simulink model "vizTest"  (R2012b)
settings: Solver=FixedStepDiscrete  StartTime=0.0  StopTime=10.0  FixedStep=0.001  RelTol=1e-3
undefined symbols (not defined in the file): clickHoldTime, clickPercentage, clickSource, cursorConstants, cursorDiameter, expRandBinSize, expRandMax, expRandMin, expRandMu, failurePenalty, gain, gloveBias, gloveIndices, gloveThreshold, hmmClickLikelihoodThreshold, holdTime, initialInput, inputType, mouseOffset, numTargets, numTrials, pbData, randomSeed, recenterDelay, recenterOnFail, recenterOnSuccess, showNeuralCursor, showScores, stopOnClick, targetDiameter, targetInds, taskType, trialsPerScore, trialTimeout, useRandomDelay, workspaceX, workspaceY
libraries: simulink x1, xpclib x1
settings Model: BufferReuse=off  Creator=gilja  LastModifiedBy=nptl
settings SolverCC: EnableConcurrentExecution=on  ConcurrentTasks=on
settings DataIOCC: SaveOutput=off  SignalLogging=off  SaveTime=off
settings OptimizationCC: InlineParams=on  InlineInvariantSignals=on  OptimizeBlockIOStorage=off  BufferReuse=off  ExpressionFolding=off  LocalBlockOutputs=off  SimCompilerOptimization=On
settings DebuggingCC: UnderspecifiedInitializationDetection=Simplified
settings HardwareCC: ProdIntDivRoundTo=Zero  ProdEndianess=LittleEndian  ProdHWDeviceType=Generic->32-bit x86 compatible
settings ModelReferenceCC: ModelReferenceNumInstancesAllowed=Single  ModelReferenceMinAlgLoopOccurrences=on
settings RTWCC: SystemTargetFile=xpctarget.tlc  TemplateMakefile=xpc_default_tmf  Description=xPC Target  ProcessScript=xpctarget_make_rtw_hook  RTWCompilerOptimization=On
settings CodeAppCC: MaxIdLength=62
settings xpcTargetCC: TargetFcnLib=ansi_tfl_table_tmw.mat  CodeReplacementLibrary=XPC_BLAS  ParMdlRefBuildCompliant=on  ConcurrentExecutionCompliant=on  CombineSignalStateStructs=off  GRTInterface=on  xPCTaskExecutionProfile=on  xPCRL32EventNumber=5000  xPCisDownloadable=off  xPCLoadParamSetFile=off  xPCConcurrentTasks=off  xPCEnableSFAnimation=off

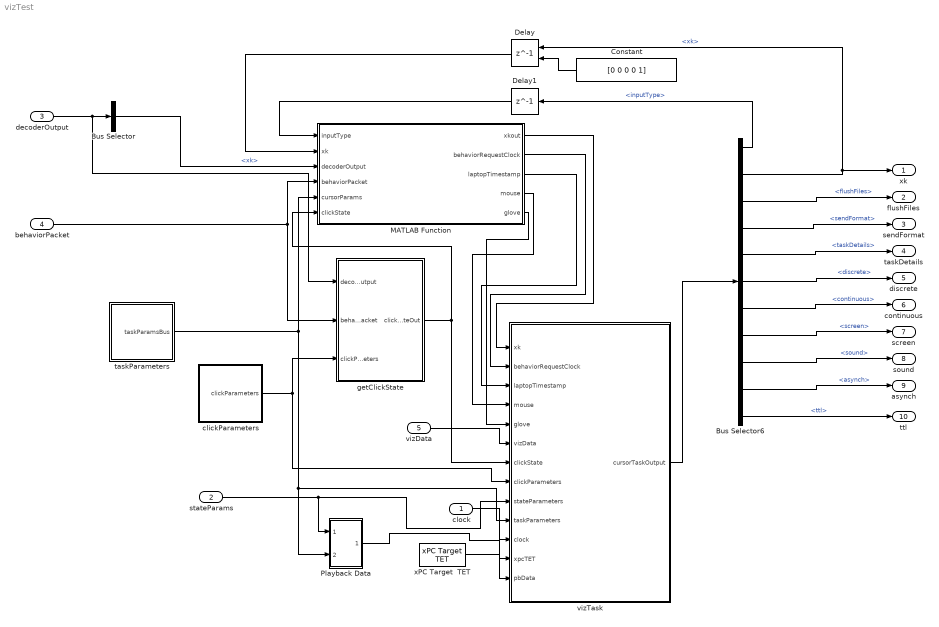
== system vizTest ==
  clock : Inport  OutDataTypeStr=uint32
  stateParams : Inport  Port=2  OutDataTypeStr=Bus: stateParams
  decoderOutput : Inport  Port=3  OutDataTypeStr=Bus: decoderOutput
  behaviorPacket : Inport  Port=4  OutDataTypeStr=Bus: behaviorPacketBus
  vizData : Inport  Port=5  OutDataTypeStr=Bus: peripheralData
  Bus Selector : BusSelector  OutputSignals=xk
  Bus Selector6 : BusSelector  OutputSignals=inputType,xk,flushFiles,sendFormat,taskDetails,discrete,continuous,screen,sound,asynch,ttl
  Constant : Constant  Value=[0 0 0 0 1]
  Delay : Delay  DelayLength=1  InitialConditionSource=Input port  InitialCondition=0
      settings: InputPortMap=u0,p4
  Delay1 : Delay  DelayLength=1  InitialCondition=0
  MATLAB Function : MATLAB Function  TreatAsAtomicUnit=on
  Playback Data : Subsystem
  clickParameters : Subsystem
  getClickState : MATLAB Function  TreatAsAtomicUnit=on
  taskParameters : Subsystem
  vizTask : MATLAB Function  TreatAsAtomicUnit=on
  "xPC Target  TET " : xpclib/Misc./xPC Target  TET   ts=0.001
  xk : Outport
  flushFiles : Outport  Port=2
  sendFormat : Outport  Port=3
  taskDetails : Outport  Port=4  OutDataTypeStr=Bus: fileLoggerFormat  BusOutputAsStruct=on
  discrete : Outport  Port=5  OutDataTypeStr=Bus: fileLoggerFormatAndData  BusOutputAsStruct=on
  continuous : Outport  Port=6  OutDataTypeStr=Bus: fileLoggerFormatAndData  BusOutputAsStruct=on
  screen : Outport  Port=7  OutDataTypeStr=Bus: fileLoggerFormatAndData  BusOutputAsStruct=on
  sound : Outport  Port=8  OutDataTypeStr=Bus: fileLoggerFormatAndData  BusOutputAsStruct=on
  asynch : Outport  Port=9  OutDataTypeStr=Bus: fileLoggerFormatAndData  BusOutputAsStruct=on
  ttl : Outport  Port=10  OutDataTypeStr=double  BusOutputAsStruct=on
  wires:
  clock/1 -> vizTask/11(clock)
  taskParameters/1(taskParamsBus) -> MATLAB Function/5(cursorParams), vizTask/10(taskParameters), Playback Data/2(cursorParams)
  "xPC Target  TET "/1 -> vizTask/12(xpcTET)
  stateParams/1 -> vizTask/9(stateParameters), Playback Data/1(stateParams)
  vizTask/1(cursorTaskOutput) -> Bus Selector6/1
  Bus Selector6/2 -> Delay/1, xk/1  "<xk>"
  Bus Selector6/3 -> flushFiles/1  "<flushFiles>"
  Bus Selector6/4 -> sendFormat/1  "<sendFormat>"
  Bus Selector6/6 -> discrete/1  "<discrete>"
  Bus Selector6/7 -> continuous/1  "<continuous>"
  Bus Selector6/5 -> taskDetails/1  "<taskDetails>"
  vizData/1 -> vizTask/6(vizData)
  MATLAB Function/1(xkout) -> vizTask/1(xk)
  Bus Selector6/8 -> screen/1  "<screen>"
  Delay/1 -> MATLAB Function/2(xk)
  MATLAB Function/2(behaviorRequestClock) -> vizTask/2(behaviorRequestClock)
  MATLAB Function/3(laptopTimestamp) -> vizTask/3(laptopTimestamp)
  MATLAB Function/4(mouse) -> vizTask/4(mouse)
  Bus Selector6/1 -> Delay1/1  "<inputType>"
  Delay1/1 -> MATLAB Function/1(inputType)
  Constant/1 -> Delay/2
  Playback Data/1(pbData) -> vizTask/13(pbData)
  behaviorPacket/1 -> MATLAB Function/4(behaviorPacket), getClickState/2(behaviorPacket)
  clickParameters/1(clickParameters) -> getClickState/3(clickParameters), vizTask/8(clickParameters)
  getClickState/1(clickStateOut) -> vizTask/7(clickState), MATLAB Function/6(clickState)
  MATLAB Function/5(glove) -> vizTask/5(glove)
  decoderOutput/1 -> getClickState/1(decoderOutput), Bus Selector/1
  Bus Selector/1 -> MATLAB Function/3(decoderOutput)  "<xk>"
  Bus Selector6/11 -> ttl/1  "<ttl>"
  Bus Selector6/9 -> sound/1  "<sound>"
  Bus Selector6/10 -> asynch/1  "<asynch>"

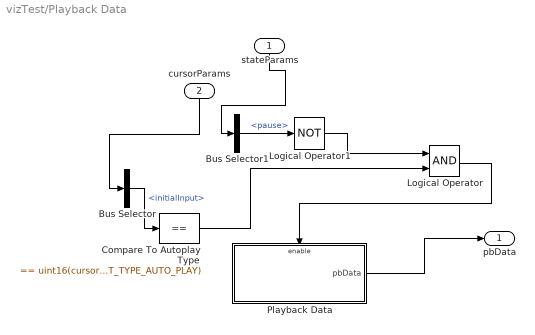
== system vizTest/Playback Data ==
  stateParams : Inport
  cursorParams : Inport  Port=2
  Bus Selector : BusSelector  OutputSignals=initialInput
  Bus Selector1 : BusSelector  OutputSignals=pause
  Compare To Autoplay Type : simulink/Logic and Bit Operations/Compare To Constant  relop===  const=uint16(cursorConstants.INPUT_TYPE_AUTO_PLAY)  OutDataTypeStr=boolean
  Logical Operator : Logic  AllPortsSameDT=off  OutDataTypeStr=boolean
  Logical Operator1 : Logic  Operator=NOT  AllPortsSameDT=off  OutDataTypeStr=boolean
  Playback Data : Subsystem
  pbData : Outport
  wires:
  Logical Operator/1 -> Playback Data/Enable
  Playback Data/1(pbData) -> pbData/1
  stateParams/1 -> Bus Selector1/1
  cursorParams/1 -> Bus Selector/1
  Bus Selector1/1 -> Logical Operator1/1  "<pause>"
  Bus Selector/1 -> Compare To Autoplay Type/1  "<initialInput>"
  Compare To Autoplay Type/1 -> Logical Operator/2
  Logical Operator1/1 -> Logical Operator/1

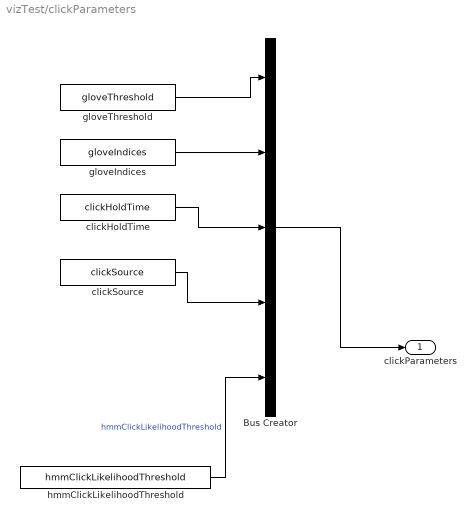
== system vizTest/clickParameters ==
  Bus Creator : BusCreator  Inputs=5  OutDataTypeStr=Bus: clickParametersBus  NonVirtualBus=on
  clickHoldTime : Constant  Value=clickHoldTime
  clickSource : Constant  Value=clickSource
  gloveIndices : Constant  Value=gloveIndices
  gloveThreshold : Constant  Value=gloveThreshold
  hmmClickLikelihoodThreshold : Constant  Value=hmmClickLikelihoodThreshold  VectorParams1D=off
  clickParameters : Outport
  wires:
  Bus Creator/1 -> clickParameters/1
  gloveThreshold/1 -> Bus Creator/1
  gloveIndices/1 -> Bus Creator/2
  clickHoldTime/1 -> Bus Creator/3
  clickSource/1 -> Bus Creator/4
  hmmClickLikelihoodThreshold/1 -> Bus Creator/5  "hmmClickLikelihoodThreshold"

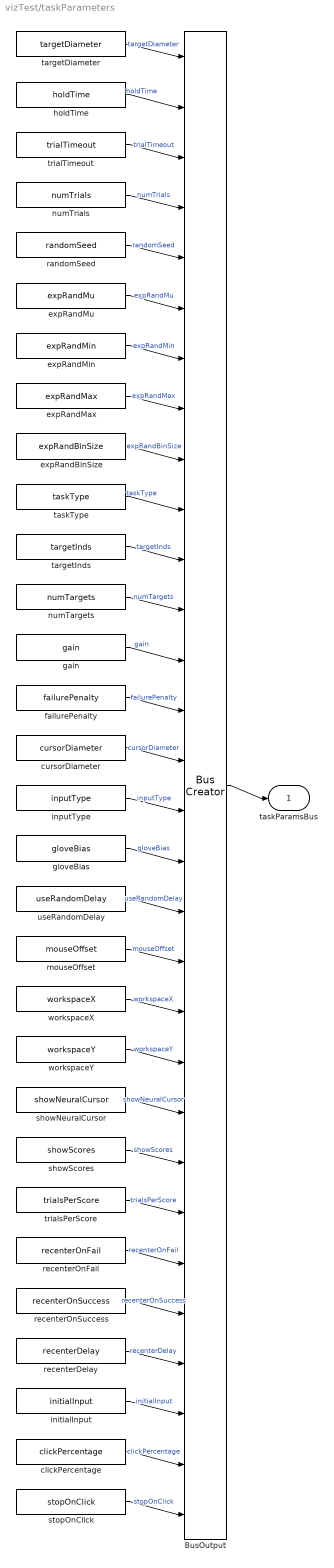
== system vizTest/taskParameters ==
  BusOutput : BusCreator  Inputs=targetDiameter,holdTime,trialTimeout,numTrials,randomSeed,expRandMu,expRandMin,expRandMax,expRandBinSize,taskType,targetInds,numTargets,gain,failurePenalty,cursorDiameter,inputType,gloveBias,useRandomDelay,mouseOffset,workspaceX,workspaceY,showNeuralCursor,showScores,trialsPerScore,recenterOnFail,recenterOnSuccess,recenterDelay,initialInput,clickPercentage,stopOnClick  OutDataTypeStr=Bus: taskParamsBus
  clickPercentage : Constant  Value=clickPercentage
  cursorDiameter : Constant  Value=cursorDiameter
  expRandBinSize : Constant  Value=expRandBinSize
  expRandMax : Constant  Value=expRandMax
  expRandMin : Constant  Value=expRandMin
  expRandMu : Constant  Value=expRandMu
  failurePenalty : Constant  Value=failurePenalty
  gain : Constant  Value=gain
  gloveBias : Constant  Value=gloveBias
  holdTime : Constant  Value=holdTime
  initialInput : Constant  Value=initialInput
  inputType : Constant  Value=inputType
  mouseOffset : Constant  Value=mouseOffset
  numTargets : Constant  Value=numTargets
  numTrials : Constant  Value=numTrials
  randomSeed : Constant  Value=randomSeed
  recenterDelay : Constant  Value=recenterDelay
  recenterOnFail : Constant  Value=recenterOnFail
  recenterOnSuccess : Constant  Value=recenterOnSuccess
  showNeuralCursor : Constant  Value=showNeuralCursor
  showScores : Constant  Value=showScores
  stopOnClick : Constant  Value=stopOnClick
  targetDiameter : Constant  Value=targetDiameter
  targetInds : Constant  Value=targetInds
  taskType : Constant  Value=taskType
  trialTimeout : Constant  Value=trialTimeout
  trialsPerScore : Constant  Value=trialsPerScore
  useRandomDelay : Constant  Value=useRandomDelay
  workspaceX : Constant  Value=workspaceX
  workspaceY : Constant  Value=workspaceY
  taskParamsBus : Outport
  wires:
  targetDiameter/1 -> BusOutput/1  "targetDiameter"
  holdTime/1 -> BusOutput/2  "holdTime"
  trialTimeout/1 -> BusOutput/3  "trialTimeout"
  numTrials/1 -> BusOutput/4  "numTrials"
  randomSeed/1 -> BusOutput/5  "randomSeed"
  expRandMu/1 -> BusOutput/6  "expRandMu"
  expRandMin/1 -> BusOutput/7  "expRandMin"
  expRandMax/1 -> BusOutput/8  "expRandMax"
  expRandBinSize/1 -> BusOutput/9  "expRandBinSize"
  taskType/1 -> BusOutput/10  "taskType"
  targetInds/1 -> BusOutput/11  "targetInds"
  numTargets/1 -> BusOutput/12  "numTargets"
  gain/1 -> BusOutput/13  "gain"
  failurePenalty/1 -> BusOutput/14  "failurePenalty"
  cursorDiameter/1 -> BusOutput/15  "cursorDiameter"
  inputType/1 -> BusOutput/16  "inputType"
  gloveBias/1 -> BusOutput/17  "gloveBias"
  useRandomDelay/1 -> BusOutput/18  "useRandomDelay"
  mouseOffset/1 -> BusOutput/19  "mouseOffset"
  workspaceX/1 -> BusOutput/20  "workspaceX"
  workspaceY/1 -> BusOutput/21  "workspaceY"
  showNeuralCursor/1 -> BusOutput/22  "showNeuralCursor"
  showScores/1 -> BusOutput/23  "showScores"
  trialsPerScore/1 -> BusOutput/24  "trialsPerScore"
  recenterOnFail/1 -> BusOutput/25  "recenterOnFail"
  recenterOnSuccess/1 -> BusOutput/26  "recenterOnSuccess"
  recenterDelay/1 -> BusOutput/27  "recenterDelay"
  initialInput/1 -> BusOutput/28  "initialInput"
  clickPercentage/1 -> BusOutput/29  "clickPercentage"
  stopOnClick/1 -> BusOutput/30  "stopOnClick"
  BusOutput/1 -> taskParamsBus/1

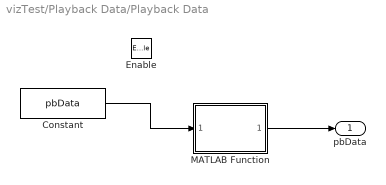
== system vizTest/Playback Data/Playback Data ==
  Enable : EnablePort
  Constant : Constant  Value=pbData
  MATLAB Function : MATLAB Function  TreatAsAtomicUnit=on
  pbData : Outport  InitialOutput=[0]
  wires:
  Constant/1 -> MATLAB Function/1(pbData)
  MATLAB Function/1(pbDataSelect) -> pbData/1

== matlab function vizTest/Playback Data/Playback Data/MATLAB Function ==
  data: pbData input single; pbDataSelect output single
function pbDataSelect = fcn(pbData)
%#codegen
persistent idx;

MAX_PLAYBACK_LENGTH = 300*1000;

if(isempty(idx))
    idx = 1;
end

pbDataSelect = pbData(idx, :);

if((idx < size(pbData,1)) && (idx < MAX_PLAYBACK_LENGTH))
    idx = idx + 1;
else
    pbDataSelect = single([0 -10000 -10000 -10000 -10000]);
end

== matlab function vizTest/MATLAB Function ==
  data: inputType input uint16 size=1; xk input size=[5 1]; decoderOutput input size=[5 1]; xkout output size=[5 1]; behaviorPacket input; cursorParams input; behaviorRequestClock output uint32 size=1; laptopTimestamp output uint8 size=16; mouse output int32 size=6; clickState input; glove output
function [xkout,behaviorRequestClock, laptopTimestamp, mouse, glove] = updateXk(inputType, xk, decoderOutput, behaviorPacket, cursorParams, clickState)


xkout = xk;

if ~cursorParams.stopOnClick || clickState == uint16(DiscreteStates.CLICK_IDLE) 
    switch inputType
        case cursorConstants.INPUT_TYPE_MOUSE_RELATIVE
            xkout(3) = cursorParams.gain(1).*double(behaviorPacket.mouse(1));
            xkout(4) = cursorParams.gain(2).*double(behaviorPacket.mouse(2));
        case cursorConstants.INPUT_TYPE_MOUSE_ABSOLUTE
            xkout(3) = cursorParams.gain(1).*(double(behaviorPacket.mouse(1))-double(cursorParams.mouseOffset(1))) - xk(1);
            xkout(4) = cursorParams.gain(2).*(double(behaviorPacket.mouse(2))-double(cursorParams.mouseOffset(2))) - xk(2);
        case cursorConstants.INPUT_TYPE_DECODE_V
            xkout(3) = decoderOutput(3);
            xkout(4) = decoderOutput(4);
    end
    xkout(1:2) = xkout(1:2)+xkout(3:4);
    if xkout(1) > cursorParams.workspaceX(2)
        xkout(1) = cursorParams.workspaceX(2);
        xkout(3) = 0;
    elseif xkout(1) < cursorParams.workspaceX(1)
        xkout(1) = cursorParams.workspaceX(1);
        xkout(3) = 0;
    end
    if xkout(2) > cursorParams.workspaceY(2)
        xkout(2) = cursorParams.workspaceY(2);
        xkout(4) = 0;
    elseif xkout(2) < cursorParams.workspaceY(1)
        xkout(2) = cursorParams.workspaceY(1);
        xkout(4) = 0;
    end
end
mouse = behaviorPacket.mouse(1:6);
glove = behaviorPacket.glove(1:5);
behaviorRequestClock = behaviorPacket.xpcRequestClock;
laptopTimestamp = behaviorPacket.laptopTimestamp(1:16);

end

== matlab function vizTest/vizTask ==
  data: xk input double size=[5 1]; behaviorRequestClock input uint32 size=1; laptopTimestamp input uint8 size=16; mouse input int32 size=6; glove input; vizData input Bus: peripheralData; clickState input; clickParameters input Bus: clickParametersBus; cursorTaskOutput output Bus: cursorTaskOutput; stateParameters input Bus: stateParams size=1; taskParameters input Bus: taskParamsBus; clock input; xpcTET input; pbData input single
function cursorTaskOutput  = vizTest(xk, behaviorRequestClock, laptopTimestamp, mouse, glove, vizData, clickState, clickParameters, stateParameters, taskParameters, clock, xpcTET, pbData)
%#codegen

%% CONSTANTS
TASK_NAME = 'viztest';
VERSION_ID = single(2.010);
NUM_DIMS = double(cursorConstants.NUM_DIMENSIONS);
STATEVEC_SIZE = 2*NUM_DIMS+1;
INIT_LENGTH = uint16(100); %ms
PRE_TRIAL_LENGTH = uint16(20); %ms
SCORE_LENGTH = uint16(4000); %ms
INIT_TIME = uint32(100);
CUE_LENGTH = taskParameters.holdTime;%uint16(200);
BLANK_LENGTH = uint16(800);


%% INITIALIZE CURSOR TASK OUTPUT
fileLoggerData.data = uint8(zeros(1,1400));
fileLoggerData.dataLen = uint16(0);
fileLoggerData.fileName = uint8(zeros(1,20));
fileLoggerData.send = false;

fileLoggerFormat.format = uint8(zeros(1,1400));
fileLoggerFormat.formatLen = uint16(0);
fileLoggerFormat.fileName = uint8(zeros(1,20));

fileLoggerFormatAndData.format = fileLoggerFormat;
fileLoggerFormatAndData.data = fileLoggerData;

cursorTaskOutput.flushFiles = false;
cursorTaskOutput.sendFormat = false;
cursorTaskOutput.taskDetails = fileLoggerFormat;
cursorTaskOutput.discrete = fileLoggerFormatAndData;
cursorTaskOutput.continuous = fileLoggerFormatAndData;
cursorTaskOutput.screen = fileLoggerFormatAndData;
cursorTaskOutput.sound = fileLoggerFormatAndData;
cursorTaskOutput.asynch = fileLoggerFormatAndData;
cursorTaskOutput.ttl = double(0);
cursorTaskOutput.xk = xk;
cursorTaskOutput.inputType = taskParameters.initialInput;

%% TASK DETAILS PACKET
cursorTaskOutput.taskDetails = packFileLoggerTaskDetails(TASK_NAME, VERSION_ID, ...
    'STATE_INIT', uint8(CursorStates.STATE_INIT), ...
    'STATE_PRE_TRIAL', uint8(CursorStates.STATE_PRE_TRIAL),...
    'STATE_NEW_TARGET', uint8(CursorStates.STATE_NEW_TARGET),...
    'STATE_MOVE', uint8(CursorStates.STATE_MOVE),...
    'STATE_ACQUIRE', uint8(CursorStates.STATE_ACQUIRE),...
    'STATE_SUCCESS', uint8(CursorStates.STATE_SUCCESS),...
    'STATE_FAIL', uint8(CursorStates.STATE_FAIL),...
    'STATE_CENTER_TARGET', uint8(CursorStates.STATE_CENTER_TARGET),...
    'STATE_END', uint8(CursorStates.STATE_END),...
    'STATE_SCORE_PAUSE', uint8(CursorStates.STATE_SCORE_PAUSE),...
    'STATE_SCORE_TARGET', uint8(CursorStates.STATE_SCORE_TARGET),...
    'STATE_RECENTER_DELAY', uint8(CursorStates.STATE_RECENTER_DELAY),...
    'STATE_MOVE_CLICK', uint8(CursorStates.STATE_MOVE_CLICK),...
    'STATE_MOVE_HOVER', uint8(CursorStates.STATE_HOVER),...
    'CLICK_IDLE', uint8(DiscreteStates.CLICK_IDLE),...
    'CLICK_MAIN', uint8(DiscreteStates.CLICK_MAIN),...
    'TASK_CENTER_OUT', uint8(cursorConstants.TASK_CENTER_OUT), ...
    'TARGET_TYPE_DWELL', uint8(cursorConstants.TARGET_TYPE_DWELL), ...
    'TARGET_TYPE_CLICK', uint8(cursorConstants.TARGET_TYPE_CLICK), ...
    'INPUT_TYPE_MOUSE_ABSOLUTE', uint8(cursorConstants.INPUT_TYPE_MOUSE_ABSOLUTE), ...
    'INPUT_TYPE_DECODE_V', uint8(cursorConstants.INPUT_TYPE_DECODE_V),...
    'INPUT_TYPE_AUTO_PLAY', uint8(cursorConstants.INPUT_TYPE_AUTO_PLAY),...
    'CLICK_TYPE_NONE', uint8(cursorConstants.CLICK_TYPE_NONE),...
    'CLICK_TYPE_GLOVE', uint8(cursorConstants.CLICK_TYPE_GLOVE),...
    'CLICK_TYPE_NEURAL', uint8(cursorConstants.CLICK_TYPE_NEURAL)...
);



%% DEFINE PERSISTENTS
persistent state vizPacket;
persistent pauseTriggered;
persistent stateTimer;
persistent holdTimer;
persistent cursorColors;

persistent currentTarget;
persistent nextTarget;
persistent currentTargetType nextTargetType;
persistent trialNum targetOrder cycleNum cycleIndex;
persistent trialDelayLength;

persistent localAcquired localTotal localTotalTime localAcqTime;
persistent localScore totalScore;
persistent acquireTime lastState;

persistent lockedParameters inputType;
persistent stateBeforePreTrial;

%% INITIALIZE PERSISTENTS
if(isempty(state))
    state = uint16(CursorStates.STATE_INIT);
    lastState = state;
    currentTarget = int16(zeros([2 1]));
    nextTarget = int16(zeros([2 1]));
    
    vizPacket = initVizPacket;
    stateTimer = uint16(0);
    holdTimer = uint16(0);
    pauseTriggered = true;
    
    cursorColors = double(zeros([3 2]));
    
    xk = double(zeros([STATEVEC_SIZE 1]));
    xk(end,1) = 1;
    
    %% buffer all the parameters off the bus
    lockedParameters = taskParameters;
    inputType = lockedParameters.initialInput;
    
    targetOrder = uint16(zeros([1 double(cursorConstants.MAX_TARGETS)]));
    trialNum = uint16(0);
    cycleNum = uint16(0);
    cycleIndex = uint16(0);
    trialDelayLength = uint16(0);
    
    localTotal = uint16(0);
    localTotalTime = uint16(0);
    localAcquired = uint16(0);
    localAcqTime = uint16(0);
    localScore = uint16(0);
    totalScore = uint16(0);
    acquireTime = stateTimer;
    currentTargetType = uint16(cursorConstants.TARGET_TYPE_DWELL);
    nextTargetType = uint16(cursorConstants.TARGET_TYPE_DWELL);
	stateBeforePreTrial = uint16(0);

end



if(clock < INIT_TIME)
    pauseTriggered = true;
end

% We usually shouldn't write discrete data
writeDiscreteData = false;
writeContinuousData = true;

if(vizData.receive && (vizData.dataLen > 0 ))
    vizPacket = parseVizPacket(vizData.data);
end

isNeural = (uint16(inputType) == uint16(cursorConstants.INPUT_TYPE_DECODE_V));
isClicked = (uint16(clickState) == uint16(DiscreteStates.CLICK_MAIN));

%% set the cursor color 
if isClicked
    cursorColors(1:end,1) = [255; 0; 0;];
else
    if isNeural
        cursorColors(1:end,1) = [255; 255; 255;];
    else
        cursorColors(1:end,1) = [255; 133; 0];
    end
end
targetColor = 'g';

%% STATE MACHINE
switch state
    case {CursorStates.STATE_INIT}
        stateTimer = stateTimer + 1;
        if stateTimer >= INIT_LENGTH
            stateTimer = uint16(0);
            state = uint16(20);
            pauseTriggered = false;
        end
        
    case 20
        cursorTaskOutput.ttl = double(1);
        stateTimer = stateTimer+1;
        if stateTimer >= CUE_LENGTH
            stateTimer = uint16(0);
            state = uint16(30);            
            cursorTaskOutput.ttl = double(0);
        end
    case 30
        cursorTaskOutput.ttl = double(0);
        stateTimer = stateTimer+1;
        if stateTimer >= BLANK_LENGTH
            stateTimer = uint16(0);
            state = uint16(20);            
            cursorTaskOutput.ttl = double(1);
        end
end

cursorTaskOutput.xk = xk;


%% PACK DATA FOR UDP OUTPUT
cursorTaskOutput.continuous = packFileLoggerFormatAndData('continuous', ...
    TASK_NAME, VERSION_ID, ...
    'clock', clock, ...
    'pause', pauseTriggered, ...
    'xpcRequestClock', behaviorRequestClock, ...
    'laptopTimestamp', laptopTimestamp, ...
    'state', state, ...
    'inputType', inputType, ...
    'mouse', mouse, ...
    'glove', glove, ...
    'laptopTimeStamp', laptopTimestamp,...
    'xpcScreenUpdateClock',vizPacket.xpcScreenUpdateClock,...
    'cursorPosition', single(xk(1:2)), ...
    'currentTarget', int16(currentTarget(:,1)), ...
    'currentTargetType', uint16(currentTargetType),...
    'clickState', uint16(clickState),...
    'xk', single(cursorTaskOutput.xk),...
    'stateTimer', stateTimer, ...
    'holdTimer', holdTimer, ...   
    'xpcTET', single(xpcTET) ...
    );




%% SEND DISCRETE DATA TO FILELOGGER
cursorTaskOutput.discrete = packFileLoggerFormatAndData('discrete', ...
    TASK_NAME, VERSION_ID, ...
    'clock', clock,...
    'state', state, ...
    'taskType', lockedParameters.taskType, ...
    'targetDiameter', lockedParameters.targetDiameter, ...
    'trialDelayLength', trialDelayLength, ...
    'gain', lockedParameters.gain, ...
    'mouseOffset', lockedParameters.mouseOffset, ...
    'cycleNum', cycleNum, ...
    'expRandMu', lockedParameters.expRandMu, ...
    'expRandMin', lockedParameters.expRandMin, ...
    'expRandMax', lockedParameters.expRandMax, ...
    'expRandBinSize', lockedParameters.expRandBinSize, ...
    'currentTarget', currentTarget,...
    'nextTarget', currentTarget,...
    'currentTargetType', uint16(currentTargetType),...
    'clickPercentage', lockedParameters.clickPercentage, ...
    'gloveThreshold', clickParameters.gloveThreshold, ...
    'gloveIndices', clickParameters.gloveIndices, ...
    'clickHoldTime', clickParameters.clickHoldTime, ...
    'clickSource', clickParameters.clickSource, ...
    'trialNum', trialNum, ...
    'trialsPerScore', lockedParameters.trialsPerScore,...
    'inputType', inputType, ...
    'showScores', lockedParameters.showScores,...
    'workspaceX', lockedParameters.workspaceX, ...
    'workspacey', lockedParameters.workspaceY, ...
    'recenterOnSuccess', lockedParameters.recenterOnSuccess,...
    'recenterOnFail', lockedParameters.recenterOnFail,...
    'recenterDelay', lockedParameters.recenterDelay,...
    'useRandomDelay', lockedParameters.useRandomDelay ...
    );

    
%% SEND DATA OUT TO VIZ
cursorTaskOutput.screen = packFileLoggerFormatAndData('screen', ...
    TASK_NAME, VERSION_ID, ...
    'clock', clock,...
    'state',state...
    ); 


%% SEND DATA OUT TO VIZ
cursorTaskOutput.sound = packFileLoggerFormatAndData('sound', ...
    TASK_NAME, VERSION_ID, ...
    'clock', clock,...
    'state',state...
    ); 


%% SET SEND FLAGS FOR NETWORK OUTPUTS
if(clock < INIT_TIME)
    cursorTaskOutput.discrete.data.send = false;
    cursorTaskOutput.continuous.data.send = false;
    cursorTaskOutput.screen.data.send = false;
    cursorTaskOutput.sound.data.send = false;
    
    if(mod(clock, 10)==0)
        cursorTaskOutput.sendFormat = true;
    else
        cursorTaskOutput.sendFormat = false;
    end
    stateTimer = uint16(0);
else
    cursorTaskOutput.discrete.data.send = writeDiscreteData;
    cursorTaskOutput.continuous.data.send = writeContinuousData;
    cursorTaskOutput.screen.data.send = true;
    cursorTaskOutput.sound.data.send = true;
    cursorTaskOutput.sendFormat = false;
    cursorTaskOutput.inputType = inputType;
end

lastState = state;

end



function vizPacket = parseVizPacket(packetData)

    vizPacket.xpcScreenUpdateClock = typecast(packetData(28+[1:4]), 'uint32');

end

function vizPacket = initVizPacket()

    vizPacket.xpcScreenUpdateClock = uint32(0);

end




function icot = isCursorOnTarget(xk, cursorRadius, targetPosition, targetRadius)
    cursorPosition = xk(1:2);
    if sqrt((double(cursorPosition(1)) - double(targetPosition(1))).^2 +...
            (double(cursorPosition(2)) - double(targetPosition(2))).^2) < double(cursorRadius+targetRadius)
        icot = true;
    else
        icot = false;
    end
    
end

== matlab function vizTest/getClickState ==
  data: decoderOutput input; behaviorPacket input Bus: behaviorPacketBus; clickStateOut output uint16; clickParameters input Bus: clickParametersBus
function clickStateOut = getClickState(decoderOutput, behaviorPacket, clickParameters)
%#codegen

persistent clickState;

if isempty(clickState)
    clickState = uint16(DiscreteStates.CLICK_IDLE);
end

clickState = uint16(DiscreteStates.CLICK_IDLE);

switch clickParameters.clickSource
    case cursorConstants.CLICK_TYPE_GLOVE
        if mean(double(behaviorPacket.glove(clickParameters.gloveIndices))) > double(clickParameters.gloveThreshold)
            clickState = uint16(DiscreteStates.CLICK_MAIN);
        end
    case cursorConstants.CLICK_TYPE_NEURAL
        if decoderOutput.clickStateLikelihood >= clickParameters.hmmClickLikelihoodThreshold
            clickState = uint16(DiscreteStates.CLICK_MAIN);
        end
end
clickStateOut = clickState;
